simulink model "rcsModelling3DOF"  (R2024a)
settings: Solver=ode45  StartTime=0.0  StopTime=100  RelTol=1e-5
PreLoadFcn:
  | run('preSimLoad.m');
InitFcn:
  | run('preSimLoad.m');
values from neighbouring files (symbols this model uses):
  gravity = 9.81    [preSimLoad.m]
  thruster_initialMass = 0.05    [preSimLoad.m]
  thrustInNewton = 10    [preSimLoad.m]
undefined symbols (not defined in the file or in its folder): aircraft, DiscIntNeverNeededParam, getCoefficient
libraries: aerolibasang x3, shared3dof x1, simulink x1
settings Model: Creator=nicol  LastModifiedBy=nicol
settings SolverCC: AlgebraicLoopSolver=TrustRegion  MinimalZcImpactIntegration=on  MaxZcPerStep=1
settings DataIOCC: SaveFormat=Array
settings OptimizationCC: EnhancedBackFolding=on  StrengthReduction=on  InitFltsAndDblsToZero=on  DifferentSizesBufferReuse=on
settings DebuggingCC: WriteAfterWriteMsg=DisableAll  AlgebraicLoopMsg=none  FcnCallInpInsideContextMsg=warning  UniqueDataStoreMsg=error  RootOutportRequireBusObject=none  StateNameClashWarn=warning  StrictBusMsg=ErrorOnBusTreatedAsVector  SFUnexpectedBacktrackingDiag=warning  SFNoUnconditionalDefaultTransitionDiag=warning  SFExecutionAtInitializationDiag=none  ArithmeticOperatorsInVariantConditions=warning
settings ModelReferenceCC: EnableRefExpFcnMdlSchedulingChecks=on  PropagateSignalLabelsOutOfModel=off
settings SFSimCC: SimUseLocalCustomCode=off
settings RTWCC: RTWUseLocalCustomCode=off  GPUComputeCapability=3.5  DLArmComputeVersion=19.05
settings CodeAppCC: StateflowObjectComments=on

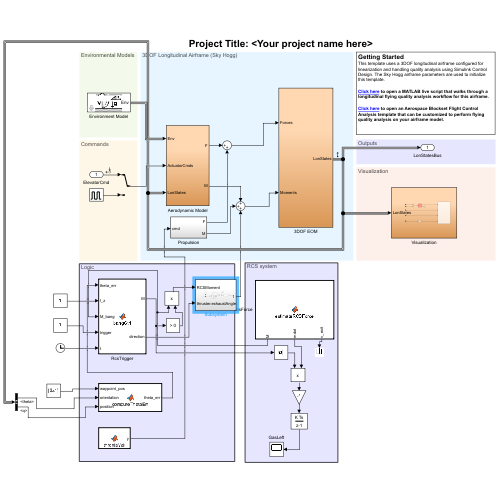
[thumbnail: Simulink's stored preview of the top-level diagram]
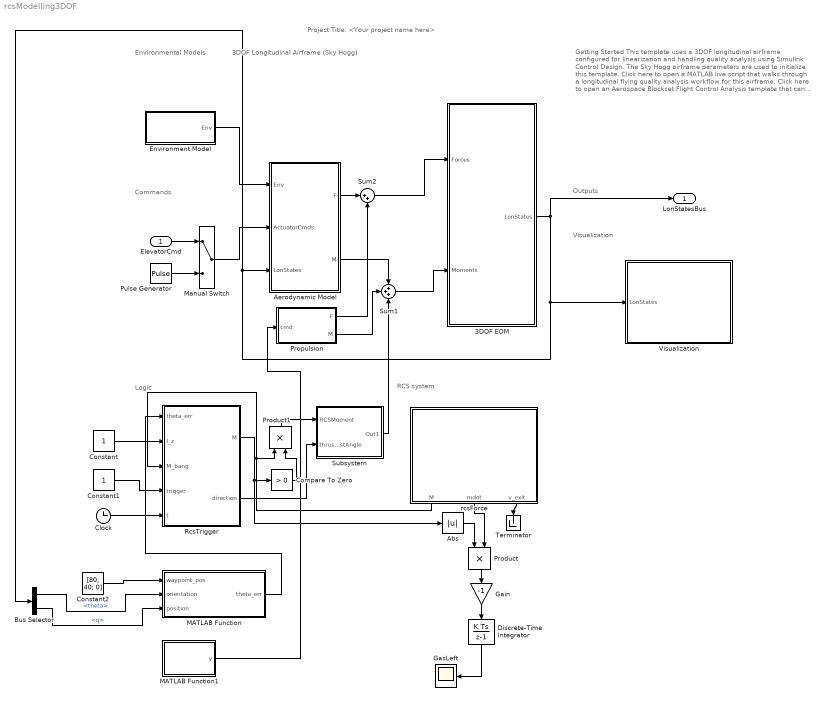
== system rcsModelling3DOF ==
  note: RCS system
  note: Logic
  note: Project Title: <Your project name here>
  note: 3DOF Longitudinal Airframe (Sky Hogg)
  note: Environmental Models
  note: Commands
  note: Visualization
  note: Outputs
  note: Getting Started
      | This template uses a 3DOF longitudinal airframe configured for linearization and handling quality analysis using Simulink Control Design. The Sky Hogg airframe parameters are used to initialize this template.
      |
      | Click here to open a MATLAB live script that walks through a longitudinal flying quality analysis workflow for this airframe.
      |
      | Click here to open an Aerospace Blockset Flight Control Analysis template that can be customized to perform flying quality analysis on your airframe model.
  ElevatorCmd : Inport
  3DOF EOM : Subsystem  VariantControl=eom3DOF
  Abs : Abs  SaturateOnIntegerOverflow=off
  Aerodynamic Model : Subsystem  VariantControl=aeroCONST
  Bus Selector : BusSelector  OutputSignals=theta,q
  Clock : Clock
  Compare To Zero : simulink/Logic and Bit Operations/Compare To Zero  relop=>  OutDataTypeStr=boolean
  Constant : Constant
  Constant1 : Constant
  Constant2 : Constant  Value=[80; 40; 0]
  Discrete-Time Integrator : DiscreteIntegrator  InitialCondition=thruster_initialMass  SampleTime=-1  ICPrevOutput=DiscIntNeverNeededParam  ICPrevScaledInput=DiscIntNeverNeededParam
  Environment Model : Subsystem  mask(Constant Environment Model){To=273, a=340, Po=101295, AirDensity=1.225, ugvgwg=[0,0,0], pgqgrg=[0,0,0], g=[0;0;gravity]}
      mask prompts: To "Constant Temperature (K):"; a "Constant Speed of Sound (m/s):"; Po "Constant Pressure (Pa):"; AirDensity "Constant Air Density (kg/m^3):"; ugvgwg "Constant Wind Velocity [ug vg wg] (m/s):"; pgqgrg "Constant Wind Angular Rates [pg qg rg] (rad/s):"; g "Constant Gravitational Acceleration (m/s^2):"
      mask Help: helpview(fullfile(docroot,'toolbox','aeroblks','aeroblks.map'), 'environment1');
      mask TypeOptions To: Constant Atmosphere/To
      mask TypeOptions a: Constant Atmosphere/a
      mask TypeOptions Po: Constant Atmosphere/Po
      mask TypeOptions AirDensity: Constant Atmosphere/AirDensity
      mask TypeOptions ugvgwg: Constant Wind/ugvgwg
      mask TypeOptions pgqgrg: Constant Wind/pgqgrg
      mask TypeOptions g: Constant Gravity/g
      mask DialogControl Container4 Prompt: Atmospheric Model
      mask DialogControl Container6 Prompt: Wind Model
      mask DialogControl Container8 Prompt: Gravity Model
      mask Display:
      | image('aeroenvironment.bmp','center')
      | port_label('output',1,'Env')
  Gain : Gain  Gain=-1
  GasLeft : Scope
  MATLAB Function : MATLAB Function  TreatAsAtomicUnit=on
  MATLAB Function1 : MATLAB Function  TreatAsAtomicUnit=on
  Manual Switch : ManualSwitch
  Product : Product
  Product1 : Product
  Propulsion : Subsystem
      settings: RTWSystemCode=Inline
  Pulse Generator : DiscretePulseGenerator  PulseType=Time based  Amplitude=-2*pi/180  Period=500  PulseWidth=.5  PhaseDelay=10
  RcsTrigger : MATLAB Function  TreatAsAtomicUnit=on
  Subsystem : Subsystem
  Sum1 : Sum  Inputs=+++  InputSameDT=on  SaturateOnIntegerOverflow=on  OutDataTypeStr=Inherit: Same as first input
  Sum2 : Sum  Inputs=|++  InputSameDT=on  SaturateOnIntegerOverflow=on  OutDataTypeStr=Inherit: Same as first input
  Terminator : Terminator
  Visualization : Subsystem
  rcsForce : MATLAB Function  TreatAsAtomicUnit=on
  LonStatesBus : Outport  VectorParamsAs1DForOutWhenUnconnected=off
  wires:
  3DOF EOM/1(LonStates) -> LonStatesBus/1, Bus Selector/1, Aerodynamic Model/3(LonStates), Visualization/1(LonStates)
  Sum2/1 -> 3DOF EOM/1(Forces)
  Propulsion/2(M) -> Sum1/2
  Propulsion/1(F) -> Sum2/2
  ElevatorCmd/1 -> Manual Switch/1
  Pulse Generator/1 -> Manual Switch/2
  Manual Switch/1 -> Aerodynamic Model/2(ActuatorCmds)
  MATLAB Function1/1(y) -> Propulsion/1(cmd)
  Sum1/1 -> 3DOF EOM/2(Moments)
  Aerodynamic Model/1(F) -> Sum2/1
  Aerodynamic Model/2(" M") -> Sum1/1
  Environment Model/1(Env) -> Aerodynamic Model/1(Env)
  rcsForce/1(M) -> RcsTrigger/3(M_bang), Product1/1
  rcsForce/3(v_exit) -> Terminator/1
  Discrete-Time Integrator/1 -> GasLeft/1
  rcsForce/2(mdot) -> Product/2
  Product/1 -> Gain/1
  Gain/1 -> Discrete-Time Integrator/1
  RcsTrigger/1(M) -> Abs/1, Compare To Zero/1
  Subsystem/1(Out1) -> Sum1/3
  Product1/1 -> Subsystem/1(RCSMoment)
  Abs/1 -> Product/1
  Compare To Zero/1 -> Product1/2
  Constant/1 -> RcsTrigger/2(I_z)
  Clock/1 -> RcsTrigger/5(t)
  Constant1/1 -> RcsTrigger/4(trigger)
  RcsTrigger/2(direction) -> Subsystem/2(thruster.exhaustAngle)
  Constant2/1 -> MATLAB Function/1(waypoint_pos)
  MATLAB Function/1(theta_err) -> RcsTrigger/1(theta_err)
  Bus Selector/1 -> MATLAB Function/2(orientation)  "<theta>"
  Bus Selector/2 -> MATLAB Function/3(position)  "<q>"

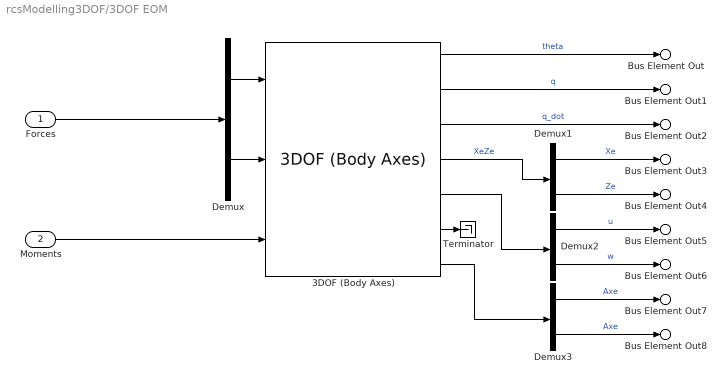
== system rcsModelling3DOF/3DOF EOM ==
  Forces : Inport
  Moments : Inport  Port=2
  3DOF (Body Axes) : shared3dof/3DOF (Body Axes)  units=Metric (MKS)  mtype=Fixed  v_ini=0  theta_ini=0  alpha_ini=0  pos_ini=[0, 0]  q_ini=0  mass=mass  mass_e=0.5  mass_f=3.0  Iyy=inertia  Iyy_e=0.5  Iyy_f=3.0  g_in=Internal  g=0  vre_flag=on  abi_flag=on  aMode=0  vel_statename={'u', 'w'}  theta_statename='theta'  pos_statename={'Xe', 'Ze'}  q_statename='q'  mass_statename=''
  Demux{,1..3} (4 alike) : Demux  Outputs=2
  Terminator : Terminator
  Bus Element Out : Outport  VectorParamsAs1DForOutWhenUnconnected=off  PortName=LonStates  Element=theta
  Bus Element Out1 : Outport  VectorParamsAs1DForOutWhenUnconnected=off  PortName=LonStates  Element=q
  Bus Element Out2 : Outport  VectorParamsAs1DForOutWhenUnconnected=off  PortName=LonStates  Element=q_dot
  Bus Element Out3 : Outport  VectorParamsAs1DForOutWhenUnconnected=off  PortName=LonStates  Element=Xe
  Bus Element Out4 : Outport  VectorParamsAs1DForOutWhenUnconnected=off  PortName=LonStates  Element=Ze
  Bus Element Out5 : Outport  VectorParamsAs1DForOutWhenUnconnected=off  PortName=LonStates  Element=u
  Bus Element Out6 : Outport  VectorParamsAs1DForOutWhenUnconnected=off  PortName=LonStates  Element=w
  Bus Element Out7 : Outport  VectorParamsAs1DForOutWhenUnconnected=off  PortName=LonStates  Element=Axe
  Bus Element Out8 : Outport  VectorParamsAs1DForOutWhenUnconnected=off  PortName=LonStates  Element=Aze
  wires:
  Demux/2 -> 3DOF (Body Axes)/2
  Demux/1 -> 3DOF (Body Axes)/1
  Forces/1 -> Demux/1
  Moments/1 -> 3DOF (Body Axes)/3
  3DOF (Body Axes)/1 -> Bus Element Out/1  "theta"
  3DOF (Body Axes)/2 -> Bus Element Out1/1  "q"
  3DOF (Body Axes)/3 -> Bus Element Out2/1  "q_dot"
  3DOF (Body Axes)/4 -> Demux1/1  "XeZe"
  3DOF (Body Axes)/5 -> Demux2/1
  3DOF (Body Axes)/7 -> Demux3/1
  Demux3/1 -> Bus Element Out7/1  "Axe"
  Demux3/2 -> Bus Element Out8/1  "Axe"
  Demux2/2 -> Bus Element Out6/1  "w"
  Demux2/1 -> Bus Element Out5/1  "u"
  Demux1/2 -> Bus Element Out4/1  "Ze"
  Demux1/1 -> Bus Element Out3/1  "Xe"
  3DOF (Body Axes)/6 -> Terminator/1

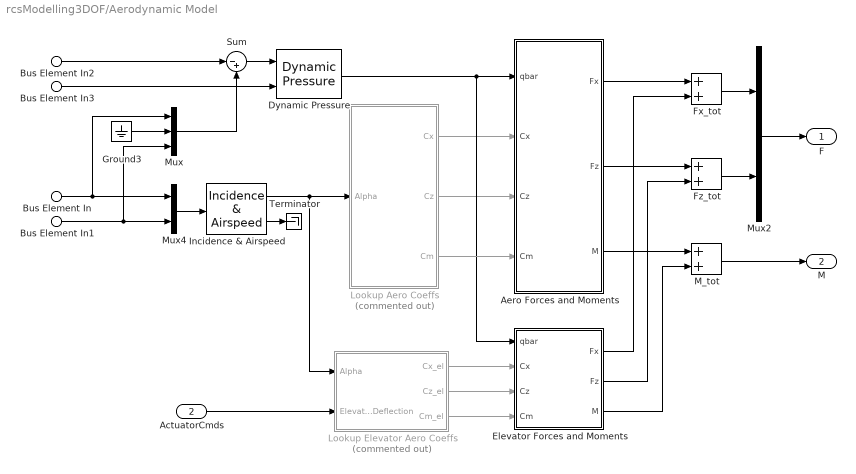
== system rcsModelling3DOF/Aerodynamic Model ==
  Bus Element In2 : Inport  PortName=Env  Element=WindVelocity
  Bus Element In3 : Inport  PortName=Env  Element=AirDensity
  ActuatorCmds : Inport  Port=2
  Bus Element In : Inport  Port=3  PortName=LonStates  Element=u
  Bus Element In1 : Inport  Port=3  PortName=LonStates  Element=w
  Aero Forces and Moments : Subsystem
  Dynamic Pressure : aerolibasang/Dynamic Pressure
  Elevator Forces and Moments : Subsystem
  Fx_tot : Sum  InputSameDT=on  SaturateOnIntegerOverflow=on  OutDataTypeStr=Inherit: Same as first input
  Fz_tot : Sum  InputSameDT=on  SaturateOnIntegerOverflow=on  OutDataTypeStr=Inherit: Same as first input
  Ground3 : Ground
  Incidence & Airspeed : aerolibasang/Incidence  & Airspeed
  Lookup Aero Coeffs : Subsystem  Commented=on
  Lookup Elevator Aero Coeffs : Subsystem  Commented=on
  M_tot : Sum  InputSameDT=on  SaturateOnIntegerOverflow=on  OutDataTypeStr=Inherit: Same as first input
  Mux : Mux  Inputs=3
  Mux2 : Mux  Inputs=2
  Mux4 : Mux  Inputs=2
  Sum : Sum  Inputs=|-+
  Terminator : Terminator
  F : Outport  VectorParamsAs1DForOutWhenUnconnected=off
  " M" : Outport  Port=2  Unit=N*m  VectorParamsAs1DForOutWhenUnconnected=off
  wires:
  Bus Element In3/1 -> Dynamic Pressure/2
  Bus Element In2/1 -> Sum/1
  Incidence & Airspeed/2 -> Terminator/1
  Bus Element In/1 -> Mux4/1, Mux/1
  Bus Element In1/1 -> Mux4/2, Mux/3
  Mux2/1 -> F/1
  Mux4/1 -> Incidence & Airspeed/1
  Ground3/1 -> Mux/2
  M_tot/1 -> " M"/1
  ActuatorCmds/1 -> Lookup Elevator Aero Coeffs/2(Elevator Deflection)
  Sum/1 -> Dynamic Pressure/1
  Incidence & Airspeed/1 -> Lookup Elevator Aero Coeffs/1(Alpha), Lookup Aero Coeffs/1(Alpha)
  Mux/1 -> Sum/2
  Elevator Forces and Moments/3(M) -> M_tot/2
  Aero Forces and Moments/1(Fx) -> Fx_tot/1
  Aero Forces and Moments/3(M) -> M_tot/1
  Elevator Forces and Moments/1(Fx) -> Fx_tot/2
  Elevator Forces and Moments/2(Fz) -> Fz_tot/2
  Aero Forces and Moments/2(Fz) -> Fz_tot/1
  Fx_tot/1 -> Mux2/1
  Fz_tot/1 -> Mux2/2
  Lookup Elevator Aero Coeffs/1(Cx_el) -> Elevator Forces and Moments/2(Cx)
  Lookup Elevator Aero Coeffs/2(Cz_el) -> Elevator Forces and Moments/3(Cz)
  Lookup Elevator Aero Coeffs/3(Cm_el) -> Elevator Forces and Moments/4(Cm)
  Lookup Aero Coeffs/2(Cz) -> Aero Forces and Moments/3(Cz)
  Lookup Aero Coeffs/1(Cx) -> Aero Forces and Moments/2(Cx)
  Dynamic Pressure/1 -> Elevator Forces and Moments/1(qbar), Aero Forces and Moments/1(qbar)
  Lookup Aero Coeffs/3(Cm) -> Aero Forces and Moments/4(Cm)

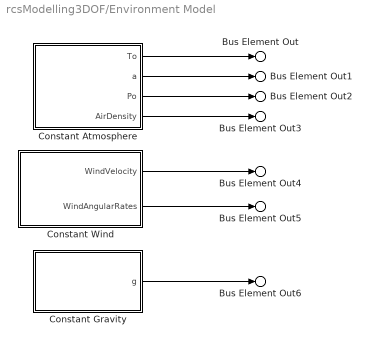
== system rcsModelling3DOF/Environment Model ==
  Constant Atmosphere : Subsystem  VariantControl=atmosCONST  mask(Standard Atmospheric Constants){To=To, a=a, Po=Po, AirDensity=AirDensity}
      mask prompts: To "Constant Temperature (K):"; a "Constant Speed of Sound (m/s):"; Po "Constant Pressure (Pa):"; AirDensity "Constant Air Density (kg/m^3):"
  Constant Gravity : Subsystem  VariantControl=gravCONST  mask(Constant Gravitational Acceleration){g=g}
      mask prompts: g "Constant Gravitational Acceleration (m/s^2):"
  Constant Wind : Subsystem  VariantControl=windCONST  mask(Constant Wind Values){ugvgwg=ugvgwg, pgqgrg=pgqgrg}
      mask prompts: ugvgwg "Constant Wind Velocity (m/s):"; pgqgrg "Constant Wind Angular Rates (rad/s):"
  Bus Element Out : Outport  VectorParamsAs1DForOutWhenUnconnected=off  PortName=Env  Element=To
  Bus Element Out1 : Outport  VectorParamsAs1DForOutWhenUnconnected=off  PortName=Env  Element=a
  Bus Element Out2 : Outport  VectorParamsAs1DForOutWhenUnconnected=off  PortName=Env  Element=Po
  Bus Element Out3 : Outport  VectorParamsAs1DForOutWhenUnconnected=off  PortName=Env  Element=AirDensity
  Bus Element Out4 : Outport  VectorParamsAs1DForOutWhenUnconnected=off  PortName=Env  Element=WindVelocity
  Bus Element Out5 : Outport  VectorParamsAs1DForOutWhenUnconnected=off  PortName=Env  Element=WindAngularRates
  Bus Element Out6 : Outport  VectorParamsAs1DForOutWhenUnconnected=off  PortName=Env  Element=g
  wires:
  Constant Wind/2(WindAngularRates) -> Bus Element Out5/1
  Constant Atmosphere/3(Po) -> Bus Element Out2/1
  Constant Atmosphere/4(AirDensity) -> Bus Element Out3/1
  Constant Atmosphere/1(To) -> Bus Element Out/1
  Constant Wind/1(WindVelocity) -> Bus Element Out4/1
  Constant Atmosphere/2(a) -> Bus Element Out1/1
  Constant Gravity/1(g) -> Bus Element Out6/1

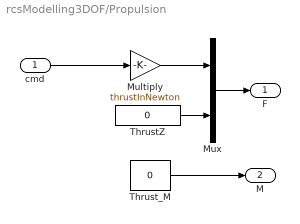
== system rcsModelling3DOF/Propulsion ==
  cmd : Inport
  Multiply : Gain  Gain=thrustInNewton
  Mux : Mux  Inputs=2
  ThrustZ : Constant  Value=0  SampleTime=-1
  Thrust_M : Constant  Value=0  SampleTime=-1
  F : Outport  Unit=N  VectorParamsAs1DForOutWhenUnconnected=off
  M : Outport  Port=2  Unit=N*m  VectorParamsAs1DForOutWhenUnconnected=off
  wires:
  Thrust_M/1 -> M/1
  Mux/1 -> F/1
  ThrustZ/1 -> Mux/2
  cmd/1 -> Multiply/1
  Multiply/1 -> Mux/1

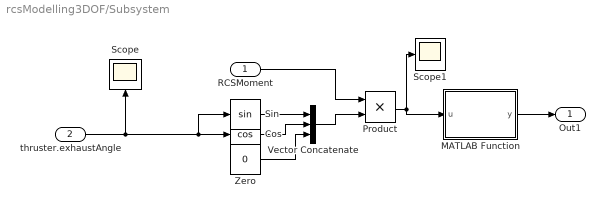
== system rcsModelling3DOF/Subsystem ==
  RCSMoment : Inport
  thruster.exhaustAngle : Inport  Port=2
  Cos : Trigonometry  Operator=cos
  MATLAB Function : MATLAB Function  TreatAsAtomicUnit=on
  Product : Product
  Scope : Scope
  Scope1 : Scope
  Sin : Trigonometry
  Vector Concatenate : Concatenate  NumInputs=3
  Zero : Constant  Value=0  OutDataTypeStr=Inherit: Inherit via back propagation
  Out1 : Outport
  wires:
  RCSMoment/1 -> Product/1
  Sin/1 -> Vector Concatenate/1
  Cos/1 -> Vector Concatenate/2
  Vector Concatenate/1 -> Product/2
  Product/1 -> Scope1/1, MATLAB Function/1(u)
  Zero/1 -> Vector Concatenate/3
  thruster.exhaustAngle/1 -> Scope/1, Sin/1, Cos/1
  MATLAB Function/1(y) -> Out1/1

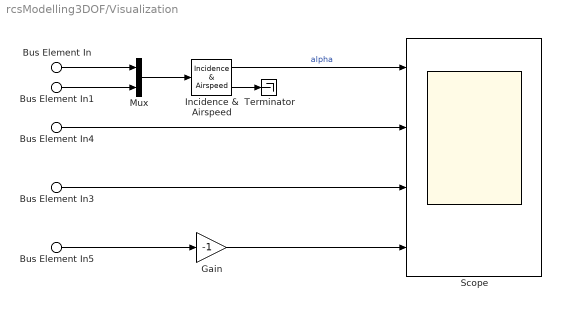
== system rcsModelling3DOF/Visualization ==
  Bus Element In : Inport  PortName=LonStates  Element=u
  Bus Element In1 : Inport  PortName=LonStates  Element=w
  Bus Element In3 : Inport  PortName=LonStates  Element=q
  Bus Element In4 : Inport  PortName=LonStates  Element=theta
  Bus Element In5 : Inport  PortName=LonStates  Element=Ze
  Gain : Gain  Gain=-1
  Incidence & Airspeed : aerolibasang/Incidence  & Airspeed
  Mux : Mux  Inputs=2
  Scope : Scope  NumInputPorts=4
  Terminator : Terminator
  wires:
  Gain/1 -> Scope/4
  Bus Element In5/1 -> Gain/1
  Bus Element In4/1 -> Scope/2
  Bus Element In3/1 -> Scope/3
  Mux/1 -> Incidence & Airspeed/1
  Bus Element In1/1 -> Mux/2
  Bus Element In/1 -> Mux/1
  Incidence & Airspeed/2 -> Terminator/1
  Incidence & Airspeed/1 -> Scope/1  "alpha"

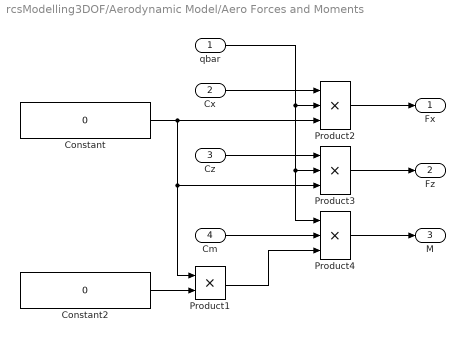
== system rcsModelling3DOF/Aerodynamic Model/Aero Forces and Moments ==
  qbar : Inport
  Cx : Inport  Port=2
  Cz : Inport  Port=3
  Cm : Inport  Port=4
  Constant : Constant  Value=0
  Constant2 : Constant  Value=0
  Product1 : Product  InputSameDT=on  SaturateOnIntegerOverflow=on  OutDataTypeStr=Inherit: Same as first input
  Product2 : Product  Inputs=3  InputSameDT=on  SaturateOnIntegerOverflow=on  OutDataTypeStr=Inherit: Same as first input
  Product3 : Product  Inputs=3  InputSameDT=on  SaturateOnIntegerOverflow=on  OutDataTypeStr=Inherit: Same as first input
  Product4 : Product  Inputs=3  InputSameDT=on  SaturateOnIntegerOverflow=on  OutDataTypeStr=Inherit: Same as first input
  Fx : Outport  VectorParamsAs1DForOutWhenUnconnected=off
  Fz : Outport  Port=2  VectorParamsAs1DForOutWhenUnconnected=off
  M : Outport  Port=3  VectorParamsAs1DForOutWhenUnconnected=off
  wires:
  Cm/1 -> Product4/2
  Product3/1 -> Fz/1
  qbar/1 -> Product4/1, Product3/2, Product2/2
  Product4/1 -> M/1
  Cx/1 -> Product2/1
  Product1/1 -> Product4/3
  Product2/1 -> Fx/1
  Cz/1 -> Product3/1
  Constant/1 -> Product1/1, Product3/3, Product2/3
  Constant2/1 -> Product1/2

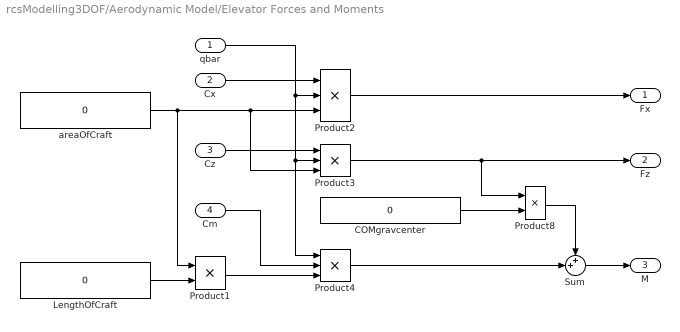
== system rcsModelling3DOF/Aerodynamic Model/Elevator Forces and Moments ==
  qbar : Inport
  Cx : Inport  Port=2
  Cz : Inport  Port=3
  Cm : Inport  Port=4
  COMgravcenter : Constant  Value=0
  LengthOfCraft : Constant  Value=0
  Product1 : Product  InputSameDT=on  SaturateOnIntegerOverflow=on  OutDataTypeStr=Inherit: Same as first input
  Product2 : Product  Inputs=3  InputSameDT=on  SaturateOnIntegerOverflow=on  OutDataTypeStr=Inherit: Same as first input
  Product3 : Product  Inputs=3  InputSameDT=on  SaturateOnIntegerOverflow=on  OutDataTypeStr=Inherit: Same as first input
  Product4 : Product  Inputs=3  InputSameDT=on  SaturateOnIntegerOverflow=on  OutDataTypeStr=Inherit: Same as first input
  Product8 : Product
  Sum : Sum  Inputs=++|
  areaOfCraft : Constant  Value=0
  Fx : Outport  VectorParamsAs1DForOutWhenUnconnected=off
  Fz : Outport  Port=2  VectorParamsAs1DForOutWhenUnconnected=off
  M : Outport  Port=3  VectorParamsAs1DForOutWhenUnconnected=off
  wires:
  COMgravcenter/1 -> Product8/2
  Product1/1 -> Product4/3
  Product8/1 -> Sum/1
  Cz/1 -> Product3/1
  Cx/1 -> Product2/1
  Product4/1 -> Sum/2
  Product2/1 -> Fx/1
  Sum/1 -> M/1
  Product3/1 -> Fz/1, Product8/1
  areaOfCraft/1 -> Product1/1, Product3/3, Product2/3
  LengthOfCraft/1 -> Product1/2
  Cm/1 -> Product4/2
  qbar/1 -> Product4/1, Product3/2, Product2/2

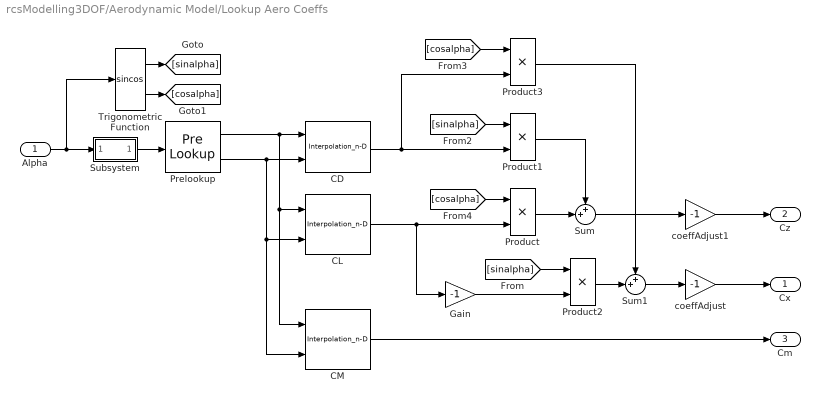
== system rcsModelling3DOF/Aerodynamic Model/Lookup Aero Coeffs ==
  Alpha : Inport  Unit=rad
  CD : Interpolation_n-D  NumberOfTableDimensions=1  Table="getCoefficient(aircraft,\"CD\",\"Zero\").Table.Value"  InternalRulePriority=Speed
      settings: InputPortMap=u0,u1
  CL : Interpolation_n-D  NumberOfTableDimensions=1  Table="getCoefficient(aircraft,\"CL\",\"Zero\").Table.Value"  InternalRulePriority=Speed
      settings: InputPortMap=u0,u1
  CM : Interpolation_n-D  NumberOfTableDimensions=1  Table="getCoefficient(aircraft,\"Cm\",\"Zero\").Table.Value"  InternalRulePriority=Speed
      settings: InputPortMap=u0,u1
  Gain : Gain  Gain=-1
  Prelookup : PreLookup  BreakpointsData="getCoefficient(aircraft,\"CD\",\"Zero\").Breakpoints(1).Value"  ExtrapMethod=Linear
  Product{,1..3} (4 alike) : Product
  Subsystem : Subsystem
      mask Display:
      | port_label('output',1,'deg')
      | port_label('input',1,'rad')
  Sum : Sum  Inputs=++|
  Sum1 : Sum  Inputs=++|
  Trigonometric Function : Trigonometry  Operator=sincos
  coeffAdjust : Gain  Gain=-1
  coeffAdjust1 : Gain  Gain=-1
  Cx : Outport  VectorParamsAs1DForOutWhenUnconnected=off
  Cz : Outport  Port=2  VectorParamsAs1DForOutWhenUnconnected=off
  Cm : Outport  Port=3  VectorParamsAs1DForOutWhenUnconnected=off
  wires:
  CL/1 -> Gain/1, Product/2
  CM/1 -> Cm/1
  Prelookup/1 -> CM/1, CL/1, CD/1
  Prelookup/2 -> CM/2, CL/2, CD/2
  Product/1 -> Sum/2
  CD/1 -> Product3/2, Product1/2
  Product1/1 -> Sum/1
  Sum/1 -> coeffAdjust1/1
  Gain/1 -> Product2/2
  Product2/1 -> Sum1/2
  Product3/1 -> Sum1/1
  Sum1/1 -> coeffAdjust/1
  coeffAdjust1/1 -> Cz/1
  coeffAdjust/1 -> Cx/1
  Alpha/1 -> Trigonometric Function/1, Subsystem/1(In1)
  [sinalpha] -> Product2/1
  [sinalpha] -> Product1/1
  [cosalpha] -> Product3/1
  [cosalpha] -> Product/1
  Trigonometric Function/2 -> [cosalpha]
  Trigonometric Function/1 -> [sinalpha]
  Subsystem/1(Out2) -> Prelookup/1

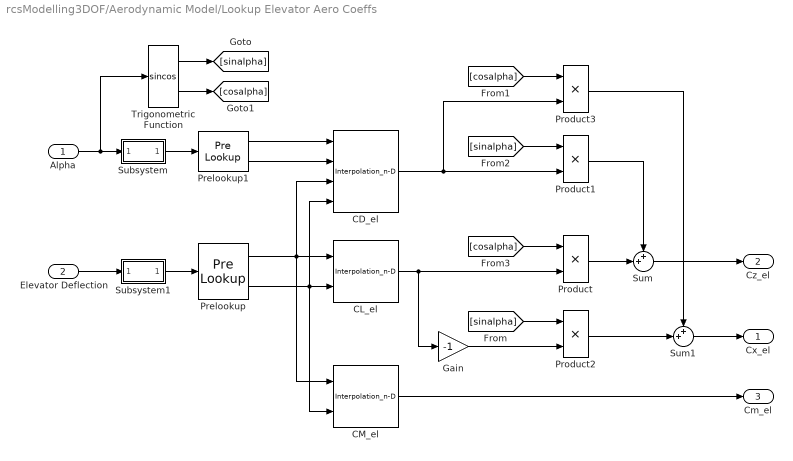
== system rcsModelling3DOF/Aerodynamic Model/Lookup Elevator Aero Coeffs ==
  Alpha : Inport  Unit=rad
  Elevator Deflection : Inport  Port=2  Unit=rad
  CD_el : Interpolation_n-D  Table="getCoefficient(aircraft,\"CD\",\"Elevator\",Component=\"Elevator\").Table.Value"
  CL_el : Interpolation_n-D  NumberOfTableDimensions=1  Table="getCoefficient(aircraft,\"CL\",\"Elevator\",Component=\"Elevator\").Table.Value"  InternalRulePriority=Speed
      settings: InputPortMap=u0,u1
  CM_el : Interpolation_n-D  NumberOfTableDimensions=1  Table="getCoefficient(aircraft,\"Cm\",\"Elevator\",Component=\"Elevator\").Table.Value"  InternalRulePriority=Speed
      settings: InputPortMap=u0,u1
  Gain : Gain  Gain=-1
  Prelookup : PreLookup  BreakpointsData="getCoefficient(aircraft,\"CD\",\"Elevator\",Component=\"Elevator\").Breakpoints(2).Value"  ExtrapMethod=Linear  IndexDataTypeStr=int32  FractionDataTypeStr=double
  Prelookup1 : PreLookup  BreakpointsData="getCoefficient(aircraft,\"CD\",\"Elevator\",Component=\"Elevator\").Breakpoints(1).Value"  ExtrapMethod=Linear  IndexDataTypeStr=int32  FractionDataTypeStr=double
  Product{,1..3} (4 alike) : Product
  Subsystem : Subsystem
      mask Display:
      | port_label('output',1,'deg')
      | port_label('input',1,'rad')
  Subsystem1 : Subsystem
      mask Display:
      | port_label('output',1,'deg')
      | port_label('input',1,'rad')
  Sum : Sum  Inputs=++|
  Sum1 : Sum  Inputs=++|
  Trigonometric Function : Trigonometry  Operator=sincos
  Cx_el : Outport  VectorParamsAs1DForOutWhenUnconnected=off
  Cz_el : Outport  Port=2  VectorParamsAs1DForOutWhenUnconnected=off
  Cm_el : Outport  Port=3  VectorParamsAs1DForOutWhenUnconnected=off
  wires:
  Sum1/1 -> Cx_el/1
  CM_el/1 -> Cm_el/1
  Sum/1 -> Cz_el/1
  Product1/1 -> Sum/1
  Product/1 -> Sum/2
  Product2/1 -> Sum1/2
  CL_el/1 -> Product/2, Gain/1
  Product3/1 -> Sum1/1
  Gain/1 -> Product2/2
  CD_el/1 -> Product1/2, Product3/2
  Prelookup/1 -> CM_el/1, CL_el/1, CD_el/3
  Prelookup/2 -> CD_el/4, CL_el/2, CM_el/2
  Alpha/1 -> Subsystem/1(In1), Trigonometric Function/1
  Subsystem/1(Out2) -> Prelookup1/1
  Elevator Deflection/1 -> Subsystem1/1(In1)
  Prelookup1/1 -> CD_el/1
  Prelookup1/2 -> CD_el/2
  [sinalpha] -> Product2/1
  [sinalpha] -> Product1/1
  [cosalpha] -> Product3/1
  [cosalpha] -> Product/1
  Trigonometric Function/2 -> [cosalpha]
  Trigonometric Function/1 -> [sinalpha]
  Subsystem1/1(Out2) -> Prelookup/1

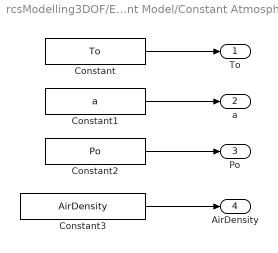
== system rcsModelling3DOF/Environment Model/Constant Atmosphere ==
  Constant : Constant  Value=To
  Constant1 : Constant  Value=a
  Constant2 : Constant  Value=Po
  Constant3 : Constant  Value=AirDensity
  To : Outport  VectorParamsAs1DForOutWhenUnconnected=off
  a : Outport  Port=2  VectorParamsAs1DForOutWhenUnconnected=off
  Po : Outport  Port=3  VectorParamsAs1DForOutWhenUnconnected=off
  AirDensity : Outport  Port=4  VectorParamsAs1DForOutWhenUnconnected=off
  wires:
  Constant1/1 -> a/1
  Constant/1 -> To/1
  Constant2/1 -> Po/1
  Constant3/1 -> AirDensity/1

== system rcsModelling3DOF/Environment Model/Constant Gravity ==
  Reshape1 : Reshape  OutputDimensionality=Column vector (2-D)
  Standard Gravity : Constant  Value=g
  g : Outport  VectorParamsAs1DForOutWhenUnconnected=off
  wires:
  Reshape1/1 -> g/1
  Standard Gravity/1 -> Reshape1/1

== system rcsModelling3DOF/Environment Model/Constant Wind ==
  Reshape : Reshape  OutputDimensionality=Column vector (2-D)
  Reshape1 : Reshape  OutputDimensionality=Column vector (2-D)
  pg,qg,rg : Constant  Value=pgqgrg
  ug,vg,wg : Constant  Value=ugvgwg
  WindVelocity : Outport  VectorParamsAs1DForOutWhenUnconnected=off
  WindAngularRates : Outport  Port=2  VectorParamsAs1DForOutWhenUnconnected=off
  wires:
  pg,qg,rg/1 -> Reshape1/1
  ug,vg,wg/1 -> Reshape/1
  Reshape/1 -> WindVelocity/1
  Reshape1/1 -> WindAngularRates/1

== system rcsModelling3DOF/Aerodynamic Model/Lookup Aero Coeffs/Subsystem ==
  In1 : Inport
  Signal Specification : SignalSpecification  Unit=deg
  Unit Conversion : UnitConversion
  Out2 : Outport  VectorParamsAs1DForOutWhenUnconnected=off
  wires:
  Signal Specification/1 -> Out2/1
  Unit Conversion/1 -> Signal Specification/1
  In1/1 -> Unit Conversion/1

== system rcsModelling3DOF/Aerodynamic Model/Lookup Elevator Aero Coeffs/Subsystem ==
  In1 : Inport
  Signal Specification : SignalSpecification  Unit=deg
  Unit Conversion : UnitConversion
  Out2 : Outport  VectorParamsAs1DForOutWhenUnconnected=off
  wires:
  Signal Specification/1 -> Out2/1
  Unit Conversion/1 -> Signal Specification/1
  In1/1 -> Unit Conversion/1

== system rcsModelling3DOF/Aerodynamic Model/Lookup Elevator Aero Coeffs/Subsystem1 ==
  In1 : Inport
  Signal Specification : SignalSpecification  Unit=deg
  Unit Conversion : UnitConversion
  Out2 : Outport  VectorParamsAs1DForOutWhenUnconnected=off
  wires:
  In1/1 -> Unit Conversion/1
  Unit Conversion/1 -> Signal Specification/1
  Signal Specification/1 -> Out2/1

== matlab function rcsModelling3DOF/RcsTrigger ==
  settings: updateMethod=DISCRETE
  data: theta_err input; M output; I_z input; M_bang input; trigger input; t input; direction output
function [M, direction] = bangCtrl(theta_err, I_z, M_bang, trigger, t)
% Bang-bang moment controller with automatic burst timing (no drift)
%
% Inputs:
%   theta_err - [3x1] rotation error vector (rad)
%   I_z       - scalar or [3x1] moment of inertia (kg·m²)
%   M_bang    - scalar: max moment magnitude to apply (N·m)
%   trigger   - boolean: rising edge trigger
%   t         - simulation time (s)
%
% Outputs:
%   M         - [3x1] moment vector to apply (N·m)
%   direction - [3x1] unit vector along theta_err (0 if no error)

persistent t_start direction_internal active dt_burst
if isempty(t_start)
    t_start = 0;
    direction_internal = [0; 0; 0];
    dt_burst = 0;
    active = false;
end

% Default outputs
M = 0;
direction = direction_internal;

% Compute error norm
norm_err = norm(theta_err);

% Rising edge: compute new burst direction and timing
if trigger && ~active && norm_err > 0
    % Unit vector direction
    direction_internal = theta_err / norm_err;

    % Effective inertia
    if isscalar(I_z)
        I_eff = I_z;
    elseif numel(I_z) == 3
        I_eff = dot(I_z(:), abs(direction_internal).^2);
    else
        error('I_z must be scalar or 3x1');
    end

    % Burst duration for symmetric bang-bang
    dt_burst = sqrt(norm_err * I_eff / M_bang);

    % Start timing
    t_start = t;
    active = true;
end

% Output current moment
if active
    tau = t - t_start;

    if tau >= 0 && tau < dt_burst
        %M =  M_bang * direction_internal;
        M =  M_bang;
    elseif tau >= dt_burst && tau < 2 * dt_burst
        %M = -M_bang * direction_internal;
        M = -M_bang;
    elseif tau >= 2 * dt_burst
        %M = [0; 0; 0];
        M = 0;
        active = false;
    end
end

% Output current direction
direction = direction_internal;

end

== matlab function rcsModelling3DOF/rcsForce ==
  data: M output; mdot output; v_exit output
function [M, mdot, v_exit] = estimateRCSForce()
% Estimates RCS thrust force using internal gas and nozzle parameters

% Parameter definition inside structured form
params.gas.pressure           = 1e6;       % Pa
params.gas.temperature        = 293.15;    % K
params.gas.gamma              = 1.3;       
params.gas.R                  = 189;       % J/kg·K

params.thruster.Cd            = 0.85;      
params.thruster.positionFromCOM = 1.0;     % m (included for completeness)

% Area of orifice
params.thruster.area = pi * (0.001 / 2)^2;

% Exit velocity (choked flow)
v_exit = sqrt( (2 * params.gas.gamma * params.gas.R * params.gas.temperature) ...
             / (params.gas.gamma + 1) );

% Mass flow rate
mdot = params.thruster.Cd * params.thruster.area * params.gas.pressure ...
     * sqrt(params.gas.gamma / (params.gas.R * params.gas.temperature)) ...
     * (2 / (params.gas.gamma + 1))^((params.gas.gamma + 1) / (2 * (params.gas.gamma - 1)));

% Thrust
M = mdot * v_exit * params.thruster.positionFromCOM;

end

== matlab function rcsModelling3DOF/MATLAB Function ==
  data: waypoint_pos input; orientation input; theta_err output; position input
function theta_err = computeThetaErr(waypoint_pos, orientation, position)
% Computes rotation error (theta_err) to point toward a 3D waypoint
%
% Inputs:
%   waypoint_pos - [3x1] target position (world)
%   position     - [3x1] current position (world)
%   orientation  - either scalar (theta_y) or [3x1] Euler angles [θx; θy; θz]
%
% Output:
%   theta_err    - [3x1] axis-angle rotation vector (rad)

% Always output 3x1 vector
theta_err = zeros(3,1);

% Direction vector from position to waypoint
r_vec = waypoint_pos(:) - position(:);
r_dir = r_vec / norm(r_vec);

% Interpret orientation
if isscalar(orientation)
    % θy: rotation around Y-axis (in 2D: yaw)
    theta_y = orientation;
    R = [cos(theta_y) 0 sin(theta_y);
         0            1 0;
        -sin(theta_y) 0 cos(theta_y)];
    
    fwd_current = R(:,1);  % body X-axis in world frame

elseif isvector(orientation) && numel(orientation) == 3
    theta = orientation(:);  % [θx; θy; θz]
    % Build 3D rotation matrix from Euler angles (XYZ convention)
    Rx = [1 0 0;
          0 cos(theta(1)) -sin(theta(1));
          0 sin(theta(1))  cos(theta(1))];
      
    Ry = [cos(theta(2))  0 sin(theta(2));
          0             1 0;
         -sin(theta(2)) 0 cos(theta(2))];
     
    Rz = [cos(theta(3)) -sin(theta(3)) 0;
          sin(theta(3))  cos(theta(3)) 0;
          0             0            1];
    
    R = Rz * Ry * Rx;
    fwd_current = R(:,1);  % body X-axis in world frame
else
    return;  % invalid input
end

% Normalize forward direction
fwd_current = fwd_current / norm(fwd_current);

% Compute rotation axis and angle to align with waypoint
axis = cross(fwd_current, r_dir);
dot_prod = dot(fwd_current, r_dir);
dot_prod = min(max(dot_prod, -1), 1);
angle = acos(dot_prod);

% Compose axis-angle result
if norm(axis) >= 1e-6 && angle ~= 0
    axis = axis / norm(axis);
    theta_err = axis * angle;
end

end

== matlab function rcsModelling3DOF/MATLAB Function1 ==
  data: y output
function y = throttleVal()

y = 0.54;

== matlab function rcsModelling3DOF/Subsystem/MATLAB Function ==
  data: u input; y output
function y = normMatrix(u)

y = sqrt(u(1)^2+u(2)^2+u(3)^2);
